simulink model "LQR_Obsever_model"  (R2023a)
settings: Solver=VariableStepAuto  StartTime=0.0  StopTime=10.0  RelTol=1e-3
undefined symbols (not defined in the file): A, B, C, D, E, K3
settings Model: Creator=z'k'x  LastModifiedBy=z'k'x

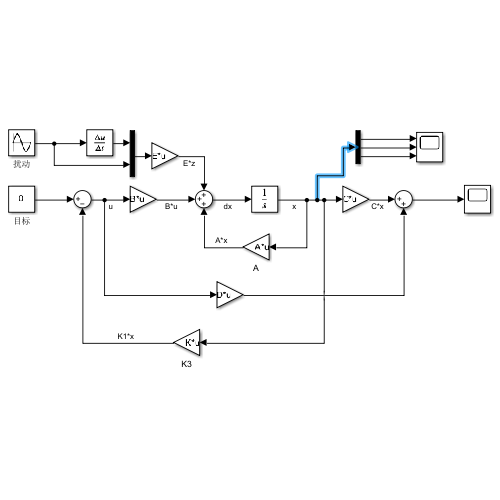
[thumbnail: Simulink's stored preview of the top-level diagram]
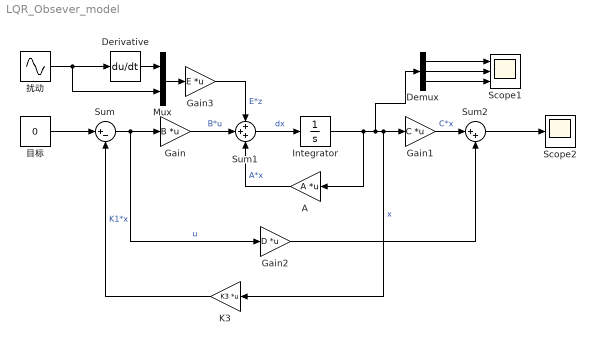
== system LQR_Obsever_model ==
  A : Gain  Gain=A  Multiplication=Matrix(K*u)
  Demux : Demux  Outputs=3
  Derivative : Derivative
  Gain : Gain  Gain=B  Multiplication=Matrix(K*u)
  Gain1 : Gain  Gain=C  Multiplication=Matrix(K*u)
  Gain2 : Gain  Gain=D  Multiplication=Matrix(K*u)
  Gain3 : Gain  Gain=E  Multiplication=Matrix(K*u)
  Integrator : Integrator
  K3 : Gain  Gain=K3  Multiplication=Matrix(K*u)
  Mux : Mux  Inputs=2
  Scope1 : Scope  NumInputPorts=3
  Scope2 : Scope
  Sum : Sum  Inputs=|+-
  Sum1 : Sum  Inputs=+++
  Sum2 : Sum  Inputs=|++
  扰动 : Sin  Frequency=17.38*2*pi  SampleTime=0
  目标 : Constant  Value=0
  wires:
  Sum2/1 -> Scope2/1
  扰动/1 -> Mux/2, Derivative/1
  Mux/1 -> Gain3/1
  Gain2/1 -> Sum2/2
  A/1 -> Sum1/3  "A*x"
  Gain/1 -> Sum1/2  "B*u"
  Sum1/1 -> Integrator/1  "dx"
  Demux/1 -> Scope1/1
  Derivative/1 -> Mux/1
  目标/1 -> Sum/1
  Sum/1 -> Gain2/1, Gain/1  "u"
  Demux/3 -> Scope1/3
  Integrator/1 -> A/1, Demux/1, K3/1, Gain1/1  "x"
  Demux/2 -> Scope1/2
  Gain3/1 -> Sum1/1  "E*z"
  K3/1 -> Sum/2  "K1*x"
  Gain1/1 -> Sum2/1  "C*x"
